simulink model "PID_Subsystem"  (R2020b)
settings: Solver=FixedStepAuto  StartTime=0.0  StopTime=120.0  FixedStep=0.001  RelTol=1e-3
settings Model: DataDictionary=Data_dictionary_prob3.sldd  Creator=Lakshmi  LastModifiedBy=Lakshmi
settings DataIOCC: SaveOutput=off  SaveTime=off

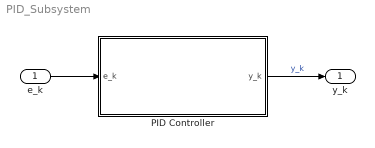
== system PID_Subsystem ==
  e_k : Inport  OutDataTypeStr=double  PortDimensions=1  SampleTime=0
  PID Controller : Subsystem  mask{Kp=370.0, Ki=50.0, Ts=0.001, Kd=-8.2490}
  y_k : Outport  OutDataTypeStr=double  PortDimensions=1  SampleTime=0
  wires:
  e_k/1 -> PID Controller/1(e_k)
  PID Controller/1(y_k) -> y_k/1  "y_k"

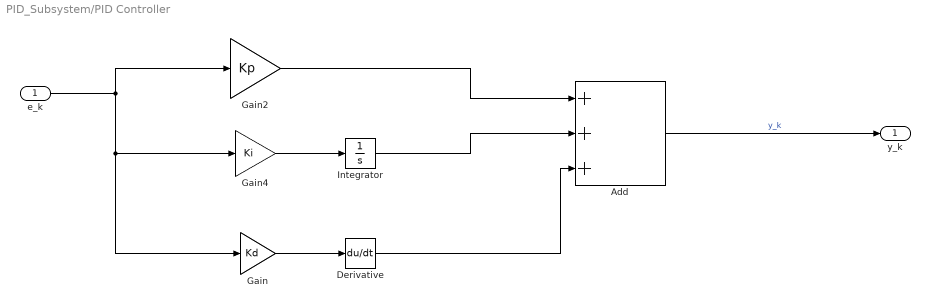
== system PID_Subsystem/PID Controller ==
  e_k : Inport
  Add : Sum  Inputs=+++
  Derivative : Derivative
  Gain : Gain  Gain=Kd
  Gain2 : Gain  Gain=Kp
  Gain4 : Gain  Gain=Ki
  Integrator : Integrator
  y_k : Outport
  wires:
  Derivative/1 -> Add/3
  Integrator/1 -> Add/2
  Gain4/1 -> Integrator/1
  Gain/1 -> Derivative/1
  Gain2/1 -> Add/1
  Add/1 -> y_k/1  "y_k"
  e_k/1 -> Gain2/1, Gain4/1, Gain/1
